simulink subsystem "GS3DX_KD_Revolute"  (R2025b)
settings: Solver=VariableStepAuto  StartTime=0.0  StopTime=10.0  RelTol=1e-3
model mask{StartPosition=0, StartVelocity=0, Dampening=0, RzPositionTargetPriority=None, RzVelocityTargetPriority=None}
  mask prompts: StartPosition "Initial Angle (deg)"; StartVelocity "Initial Angular Velocity (deg/s)"; Dampening "Dampening (N*m/(deg/s))"; RzPositionTargetPriority "Position Target Priority"; RzVelocityTargetPriority "Velocity Target Priority"
undefined symbols (not defined in the file): DampeningGlobalGain, LocalDampeningEnable
libraries: nesl_utility x14, fl_lib x3, sm_lib x3
settings Model: Creator=diete  LastModifiedBy=diete

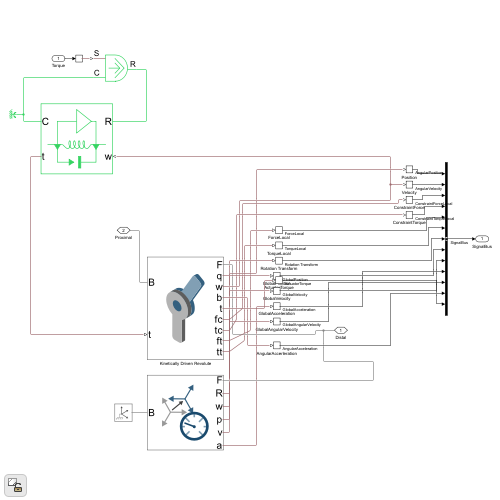
[thumbnail: Simulink's stored preview of the top-level diagram]
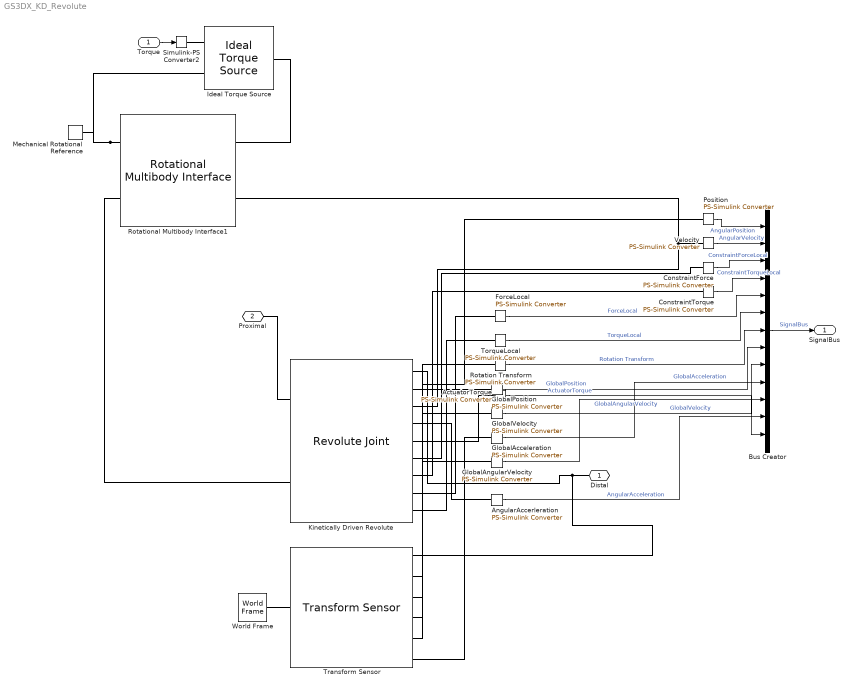
== system GS3DX_KD_Revolute ==
  Torque : Inport
  ActuatorTorque : nesl_utility/PS-Simulink Converter  PhysicalDomain=network_engine_domain  SubClassName=ps_output  LeftPortType=input  RightPortType=output  PseudoPeriodic=off  Frequencies=[]  VectorFormat=1-D array  Unit=N*m  AffineConversion=off
  AngularAccerleration : nesl_utility/PS-Simulink Converter  PhysicalDomain=network_engine_domain  SubClassName=ps_output  LeftPortType=input  RightPortType=output  PseudoPeriodic=off  Frequencies=[]  VectorFormat=1-D array  Unit=deg/s^2  AffineConversion=off
  Bus Creator : BusCreator  Inputs=13
  ConstraintForce : nesl_utility/PS-Simulink Converter  PhysicalDomain=network_engine_domain  SubClassName=ps_output  LeftPortType=input  RightPortType=output  PseudoPeriodic=off  Frequencies=[]  VectorFormat=1-D array  Unit=inherit  AffineConversion=off
  ConstraintTorque : nesl_utility/PS-Simulink Converter  PhysicalDomain=network_engine_domain  SubClassName=ps_output  LeftPortType=input  RightPortType=output  PseudoPeriodic=off  Frequencies=[]  VectorFormat=1-D array  Unit=inherit  AffineConversion=off
  ForceLocal : nesl_utility/PS-Simulink Converter  PhysicalDomain=network_engine_domain  SubClassName=ps_output  LeftPortType=input  RightPortType=output  PseudoPeriodic=off  Frequencies=[]  VectorFormat=1-D array  Unit=inherit  AffineConversion=off
  GlobalAcceleration : nesl_utility/PS-Simulink Converter  PhysicalDomain=network_engine_domain  SubClassName=ps_output  LeftPortType=input  RightPortType=output  PseudoPeriodic=off  Frequencies=[]  VectorFormat=1-D array  Unit=inherit  AffineConversion=off
  GlobalAngularVelocity : nesl_utility/PS-Simulink Converter  PhysicalDomain=network_engine_domain  SubClassName=ps_output  LeftPortType=input  RightPortType=output  PseudoPeriodic=off  Frequencies=[]  VectorFormat=1-D array  Unit=deg/s  AffineConversion=off
  GlobalPosition : nesl_utility/PS-Simulink Converter  PhysicalDomain=network_engine_domain  SubClassName=ps_output  LeftPortType=input  RightPortType=output  PseudoPeriodic=off  Frequencies=[]  VectorFormat=1-D array  Unit=inherit  AffineConversion=off
  GlobalVelocity : nesl_utility/PS-Simulink Converter  PhysicalDomain=network_engine_domain  SubClassName=ps_output  LeftPortType=input  RightPortType=output  PseudoPeriodic=off  Frequencies=[]  VectorFormat=1-D array  Unit=inherit  AffineConversion=off
  Ideal Torque Source : fl_lib/Mechanical/Mechanical Sources/Ideal Torque Source
  Kinetically Driven Revolute : sm_lib/Joints/Revolute Joint  JointMode=Normal  CompositeWrenchDir=BaseOnFollower  CompositeWrenchFrame=FollowerFrame  SenseConstraintForce=on  SenseConstraintTorque=on  SenseTotalForce=on  SenseTotalTorque=on  PositionTargetSpecify=off  PositionTargetPriority=Low  PositionTargetValue=StartPosition  PositionTargetValueUnits=deg  VelocityTargetSpecify=off  VelocityTargetPriority=Low  VelocityTargetValue=StartVelocity  VelocityTargetValueUnits=deg/s  EquilibriumPosition=0  EquilibriumPositionUnits=deg  SpringStiffness=0  SpringStiffnessUnits=N*m/deg  DampingCoefficient=Dampening*LocalDampeningEnable*DampeningGlobalGain  DampingCoefficientUnits=N*m/(deg/s)  LowerLimitSpecify=off  LowerLimitBound=-120  LowerLimitBoundUnits=deg  LowerLimitStiffness=20  LowerLimitStiffnessUnits=N*m/deg  LowerLimitDamping=0  LowerLimitDampingUnits=N*m/(deg/s)  LowerLimitTransitionRegionWidth=0.1  LowerLimitTransitionRegionWidthUnits=deg  UpperLimitSpecify=off  UpperLimitBound=0  UpperLimitBoundUnits=deg  UpperLimitStiffness=100  UpperLimitStiffnessUnits=N*m/deg  UpperLimitDamping=10  UpperLimitDampingUnits=N*m/(deg/s)  UpperLimitTransitionRegionWidth=0.1  UpperLimitTransitionRegionWidthUnits=deg  TorqueActuationMode=InputTorque  MotionActuationMode=ComputedMotion  SensePosition=on  SenseVelocity=on  SenseAcceleration=on  SenseTorqueForce=on  SenseLowerLimitTorqueForce=off  SenseUpperLimitTorqueForce=off
      settings: LogSimulationData=on
  Mechanical Rotational Reference : fl_lib/Mechanical/Rotational Elements/Mechanical Rotational Reference
  Position : nesl_utility/PS-Simulink Converter  PhysicalDomain=network_engine_domain  SubClassName=ps_output  LeftPortType=input  RightPortType=output  PseudoPeriodic=off  Frequencies=[]  VectorFormat=1-D array  Unit=deg  AffineConversion=off
  Rotation Transform : nesl_utility/PS-Simulink Converter  PhysicalDomain=network_engine_domain  SubClassName=ps_output  LeftPortType=input  RightPortType=output  PseudoPeriodic=off  Frequencies=[]  VectorFormat=1-D array  Unit=inherit  AffineConversion=off
  Rotational Multibody Interface1 : fl_lib/Mechanical/Multibody Interfaces/Rotational Multibody Interface
  Simulink-PS Converter2 : nesl_utility/Simulink-PS Converter  PhysicalDomain=network_engine_domain  SubClassName=ps_input  LeftPortType=input  RightPortType=output  PseudoPeriodic=off  Frequencies=[]  NoiseDistribution=none  NoiseParameters=[]  Unit=1  AffineConversion=off  FilteringAndDerivatives=provide  SimscapeFilterOrder=1  InputFilterTimeConstant=0.001  UdotUserProvided=0
  TorqueLocal : nesl_utility/PS-Simulink Converter  PhysicalDomain=network_engine_domain  SubClassName=ps_output  LeftPortType=input  RightPortType=output  PseudoPeriodic=off  Frequencies=[]  VectorFormat=1-D array  Unit=inherit  AffineConversion=off
  Transform Sensor : sm_lib/Frames and Transforms/Transform Sensor  MeasurementFrame=World  RotationSequence=XYX  SenseAngle=off  SenseAxis=off  SenseQ=off  SenseR=on  SenseRotationSequence=off  SenseOmegaX=off  SenseOmegaY=off  SenseOmegaZ=off  SenseOmega=on  SenseQDot=off  SenseRDot=off  SenseRotationSequenceDot=off  SenseAlphaX=off  SenseAlphaY=off  SenseAlphaZ=off  SenseAlpha=off  SenseQDDot=off  SenseRDDot=off  SenseX=off  SenseY=off  SenseZ=off  SenseXYZ=on  SenseRad=off  SenseAzim=off  SenseDist=off  SenseInc=off  SenseXDot=off  SenseYDot=off  SenseZDot=off  SenseXYZDot=on  SenseRadDot=off  SenseAzimDot=off  SenseDistDot=off  SenseIncDot=off  SenseXDDot=off  SenseYDDot=off  SenseZDDot=off  SenseXYZDDot=on  SenseRadDDot=off  SenseAzimDDot=off  SenseDistDDot=off  SenseIncDDot=off
  Velocity : nesl_utility/PS-Simulink Converter  PhysicalDomain=network_engine_domain  SubClassName=ps_output  LeftPortType=input  RightPortType=output  PseudoPeriodic=off  Frequencies=[]  VectorFormat=1-D array  Unit=deg/s  AffineConversion=off
  World Frame : sm_lib/Frames and Transforms/World Frame
  Distal : PMIOPort  Side=Right
  Proximal : PMIOPort  Port=2  Side=Left
  SignalBus : Outport
  wires:
  Position/1 -> Bus Creator/1  "AngularPosition"
  Bus Creator/1 -> SignalBus/1  "SignalBus"
  TorqueLocal/1 -> Bus Creator/6  "TorqueLocal"
  ForceLocal/1 -> Bus Creator/5  "ForceLocal"
  ConstraintForce/1 -> Bus Creator/3  "ConstraintForceLocal"
  ConstraintTorque/1 -> Bus Creator/4  "ConstraintTorqueLocal"
  Rotation Transform/1 -> Bus Creator/7  "Rotation Transform"
  GlobalPosition/1 -> Bus Creator/8  "GlobalPosition"
  GlobalVelocity/1 -> Bus Creator/9  "GlobalVelocity"
  GlobalAcceleration/1 -> Bus Creator/10  "GlobalAcceleration"
  Velocity/1 -> Bus Creator/2  "AngularVelocity"
  GlobalAngularVelocity/1 -> Bus Creator/11  "GlobalAngularVelocity"
  Torque/1 -> Simulink-PS Converter2/1
  AngularAccerleration/1 -> Bus Creator/12  "AngularAcceleration"
  ActuatorTorque/1 -> Bus Creator/13  "ActuatorTorque"
  connections:
  Distal/RConn1 -- Kinetically Driven Revolute/RConn1 -- Transform Sensor/RConn1
  Rotational Multibody Interface1/LConn2 -- Ideal Torque Source/RConn2 -- Mechanical Rotational Reference/LConn1
  Rotational Multibody Interface1/RConn1 -- Kinetically Driven Revolute/RConn3 -- Velocity/LConn1
  Proximal/RConn1 -- Kinetically Driven Revolute/LConn1
  ForceLocal/LConn1 -- Kinetically Driven Revolute/RConn8
  TorqueLocal/LConn1 -- Kinetically Driven Revolute/RConn9
  Position/LConn1 -- Kinetically Driven Revolute/RConn2
  ConstraintForce/LConn1 -- Kinetically Driven Revolute/RConn6
  ConstraintTorque/LConn1 -- Kinetically Driven Revolute/RConn7
  Transform Sensor/RConn6 -- GlobalAcceleration/LConn1
  Transform Sensor/RConn2 -- Rotation Transform/LConn1
  Transform Sensor/RConn4 -- GlobalPosition/LConn1
  Transform Sensor/RConn5 -- GlobalVelocity/LConn1
  World Frame/RConn1 -- Transform Sensor/LConn1
  Rotational Multibody Interface1/LConn1 -- Kinetically Driven Revolute/LConn2
  Transform Sensor/RConn3 -- GlobalAngularVelocity/LConn1
  Simulink-PS Converter2/RConn1 -- Ideal Torque Source/RConn1
  Ideal Torque Source/LConn1 -- Rotational Multibody Interface1/RConn2
  Kinetically Driven Revolute/RConn4 -- AngularAccerleration/LConn1
  Kinetically Driven Revolute/RConn5 -- ActuatorTorque/LConn1
